simulink model "RMCHardwareInterfaceTUM_SiL"  (R2018b)
settings: configuration reference "Active" (kept outside this file)
undefined symbols (not defined in the file): PX2_Perception_IP_1, PX2_Perception_IP_2, PX2_Perception_IP_3, PX2_Perception_IP_4, PX2_Strategy_IP_1, PX2_Strategy_IP_2, PX2_Strategy_IP_3, PX2_Strategy_IP_4
libraries: dspnetwork x12
settings Model: DataDictionary=RMCHardwareInterfaceTUM_SiL.sldd  xpc_rtwmakecfg_data=_xpcetherlib__xpcether8255xlib__xpcetherGbElib__xpcnblib__xpciplib_  Creator=wischnewski  LastModifiedBy=ge34qer

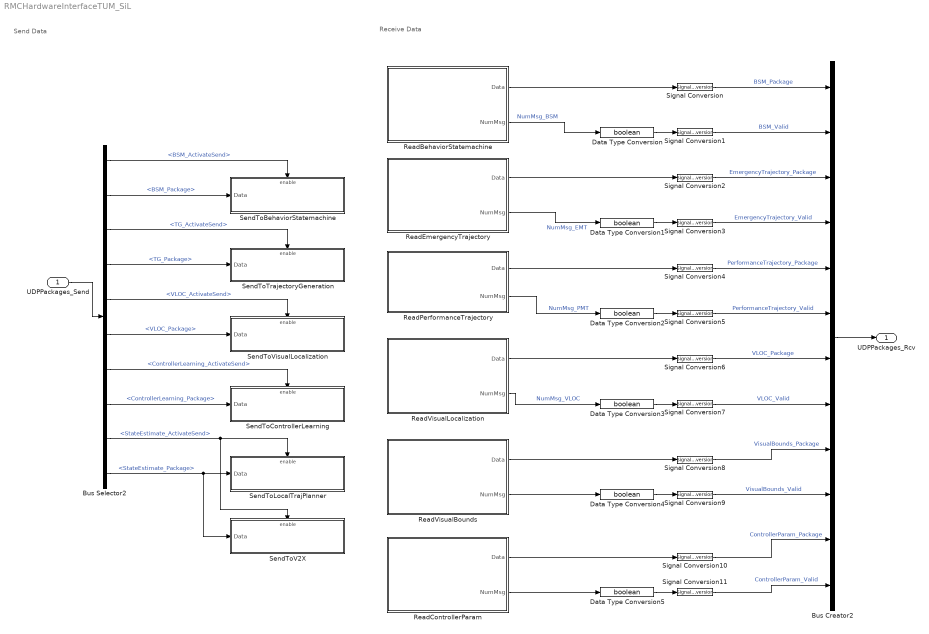
== system RMCHardwareInterfaceTUM_SiL ==
  note: Send Data
  note: Receive Data
  UDPPackages_Send : Inport  OutDataTypeStr=Bus: UDPPackages_Send
  Bus Creator2 : BusCreator  Inputs=12
  Bus Selector2 : BusSelector  OutputSignals=BSM_ActivateSend,BSM_Package,TG_ActivateSend,TG_Package,VLOC_ActivateSend,VLOC_Package,ControllerLearning_ActivateSend,ControllerLearning_Package,StateEstimate_ActivateSend,StateEstimate_Package
  Data Type Conversion{,1..5} (6 alike) : DataTypeConversion  OutDataTypeStr=boolean
  ReadBehaviorStatemachine : Subsystem  Priority=1000
  ReadControllerParam : Subsystem  Priority=1000
  ReadEmergencyTrajectory : Subsystem  Priority=1000
  ReadPerformanceTrajectory : Subsystem  Priority=1000
  ReadVisualBounds : Subsystem  Priority=1000
  ReadVisualLocalization : Subsystem  Priority=1000
  SendToBehaviorStatemachine : Subsystem
  SendToControllerLearning : Subsystem
  SendToLocalTrajPlanner : Subsystem
  SendToTrajectoryGeneration : Subsystem
  SendToV2X : Subsystem
  SendToVisualLocalization : Subsystem
  Signal Conversion{,1..11} (12 alike) : SignalConversion  OverrideOpt=off
  UDPPackages_Rcv : Outport  OutDataTypeStr=Bus: UDPPackages_Rcv
  wires:
  UDPPackages_Send/1 -> Bus Selector2/1
  Bus Selector2/2 -> SendToBehaviorStatemachine/1(Data)  "<BSM_Package>"
  Bus Selector2/1 -> SendToBehaviorStatemachine/Enable  "<BSM_ActivateSend>"
  Bus Selector2/4 -> SendToTrajectoryGeneration/1(Data)  "<TG_Package>"
  Bus Selector2/3 -> SendToTrajectoryGeneration/Enable  "<TG_ActivateSend>"
  Bus Selector2/6 -> SendToVisualLocalization/1(Data)  "<VLOC_Package>"
  Bus Selector2/5 -> SendToVisualLocalization/Enable  "<VLOC_ActivateSend>"
  Signal Conversion/1 -> Bus Creator2/1  "BSM_Package"
  Signal Conversion1/1 -> Bus Creator2/2  "BSM_Valid"
  Signal Conversion3/1 -> Bus Creator2/4  "EmergencyTrajectory_Valid"
  Signal Conversion2/1 -> Bus Creator2/3  "EmergencyTrajectory_Package"
  Signal Conversion4/1 -> Bus Creator2/5  "PerformanceTrajectory_Package"
  Signal Conversion5/1 -> Bus Creator2/6  "PerformanceTrajectory_Valid"
  Signal Conversion6/1 -> Bus Creator2/7  "VLOC_Package"
  Signal Conversion7/1 -> Bus Creator2/8  "VLOC_Valid"
  ReadVisualLocalization/1(Data) -> Signal Conversion6/1
  ReadBehaviorStatemachine/1(Data) -> Signal Conversion/1
  Data Type Conversion/1 -> Signal Conversion1/1
  ReadEmergencyTrajectory/1(Data) -> Signal Conversion2/1
  Data Type Conversion2/1 -> Signal Conversion5/1
  ReadPerformanceTrajectory/1(Data) -> Signal Conversion4/1
  Bus Creator2/1 -> UDPPackages_Rcv/1
  ReadBehaviorStatemachine/2(NumMsg) -> Data Type Conversion/1  "NumMsg_BSM"
  ReadEmergencyTrajectory/2(NumMsg) -> Data Type Conversion1/1  "NumMsg_EMT"
  ReadPerformanceTrajectory/2(NumMsg) -> Data Type Conversion2/1  "NumMsg_PMT"
  ReadVisualLocalization/2(NumMsg) -> Data Type Conversion3/1  "NumMsg_VLOC"
  Data Type Conversion1/1 -> Signal Conversion3/1
  Data Type Conversion3/1 -> Signal Conversion7/1
  ReadVisualBounds/1(Data) -> Signal Conversion8/1
  Data Type Conversion4/1 -> Signal Conversion9/1
  ReadVisualBounds/2(NumMsg) -> Data Type Conversion4/1
  Signal Conversion8/1 -> Bus Creator2/9  "VisualBounds_Package"
  Signal Conversion9/1 -> Bus Creator2/10  "VisualBounds_Valid"
  Data Type Conversion5/1 -> Signal Conversion11/1
  ReadControllerParam/1(Data) -> Signal Conversion10/1
  ReadControllerParam/2(NumMsg) -> Data Type Conversion5/1
  Signal Conversion10/1 -> Bus Creator2/11  "ControllerParam_Package"
  Signal Conversion11/1 -> Bus Creator2/12  "ControllerParam_Valid"
  Bus Selector2/7 -> SendToControllerLearning/Enable  "<ControllerLearning_ActivateSend>"
  Bus Selector2/8 -> SendToControllerLearning/1(Data)  "<ControllerLearning_Package>"
  Bus Selector2/10 -> SendToV2X/1(Data), SendToLocalTrajPlanner/1(Data)  "<StateEstimate_Package>"
  Bus Selector2/9 -> SendToV2X/Enable, SendToLocalTrajPlanner/Enable  "<StateEstimate_ActivateSend>"

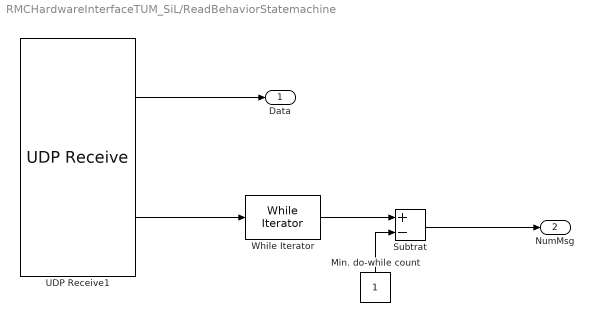
== system RMCHardwareInterfaceTUM_SiL/ReadBehaviorStatemachine ==
  Min. do-while count : Constant  OutDataTypeStr=int8
  Subtrat : Sum  Inputs=+-
  UDP Receive1 : dspnetwork/UDP Receive  localURL='0.0.0.0'  localPort=BehaviorStatemachineRcv_Port  remoteURL='0.0.0.0'  remotePort=-1  recvBufferSize=8192  dims=4  signalDatatype=uint8  isVarSize=off  showBlockingTime=on  blockingTime=0  sampletime=-1  blockPlatform=HOST
      settings: SourceProductName=DSP System Toolbox  SourceProductBaseCode=DS
  While Iterator : WhileIterator  MaxIters=-1  WhileBlockType=do-while  ShowIterationPort=on  OutputDataType=int16
  Data : Outport
  NumMsg : Outport  Port=2
  wires:
  While Iterator/1 -> Subtrat/1
  Min. do-while count/1 -> Subtrat/2
  Subtrat/1 -> NumMsg/1
  UDP Receive1/2 -> While Iterator/1
  UDP Receive1/1 -> Data/1

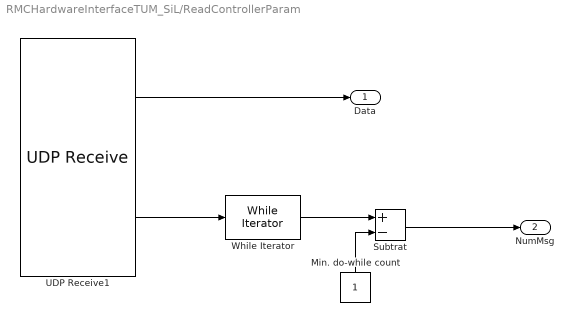
== system RMCHardwareInterfaceTUM_SiL/ReadControllerParam ==
  Min. do-while count : Constant  OutDataTypeStr=int8
  Subtrat : Sum  Inputs=+-
  UDP Receive1 : dspnetwork/UDP Receive  localURL='0.0.0.0'  localPort=ControllerParamRcv_Port  remoteURL='0.0.0.0'  remotePort=-1  recvBufferSize=8192  dims=1019  signalDatatype=uint8  isVarSize=off  showBlockingTime=on  blockingTime=0  sampletime=-1  blockPlatform=HOST
      settings: SourceProductName=DSP System Toolbox  SourceProductBaseCode=DS
  While Iterator : WhileIterator  MaxIters=-1  WhileBlockType=do-while  ShowIterationPort=on  OutputDataType=int16
  Data : Outport
  NumMsg : Outport  Port=2
  wires:
  UDP Receive1/2 -> While Iterator/1
  While Iterator/1 -> Subtrat/1
  Min. do-while count/1 -> Subtrat/2
  UDP Receive1/1 -> Data/1
  Subtrat/1 -> NumMsg/1

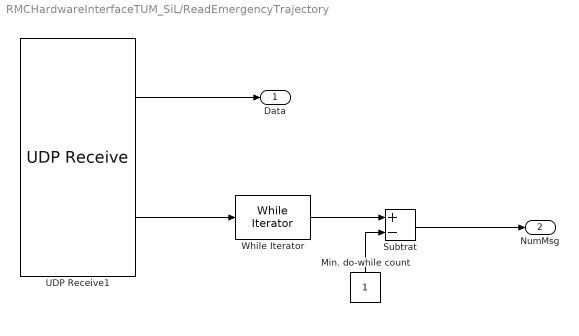
== system RMCHardwareInterfaceTUM_SiL/ReadEmergencyTrajectory ==
  Min. do-while count : Constant  OutDataTypeStr=int8
  Subtrat : Sum  Inputs=+-
  UDP Receive1 : dspnetwork/UDP Receive  localURL='0.0.0.0'  localPort=EmergencyPathRcv_Port  remoteURL='0.0.0.0'  remotePort=-1  recvBufferSize=8192  dims=1412  signalDatatype=uint8  isVarSize=off  showBlockingTime=on  blockingTime=0  sampletime=-1  blockPlatform=HOST
      settings: SourceProductName=DSP System Toolbox  SourceProductBaseCode=DS
  While Iterator : WhileIterator  MaxIters=-1  WhileBlockType=do-while  ShowIterationPort=on  OutputDataType=int16
  Data : Outport
  NumMsg : Outport  Port=2
  wires:
  While Iterator/1 -> Subtrat/1
  Min. do-while count/1 -> Subtrat/2
  UDP Receive1/2 -> While Iterator/1
  UDP Receive1/1 -> Data/1
  Subtrat/1 -> NumMsg/1

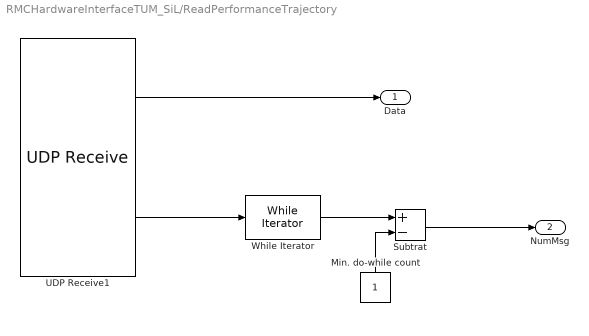
== system RMCHardwareInterfaceTUM_SiL/ReadPerformanceTrajectory ==
  Min. do-while count : Constant  OutDataTypeStr=int8
  Subtrat : Sum  Inputs=+-
  UDP Receive1 : dspnetwork/UDP Receive  localURL='0.0.0.0'  localPort=PerformanceTrajectoryRcv_Port  remoteURL='0.0.0.0'  remotePort=-1  recvBufferSize=8192  dims=1412  signalDatatype=uint8  isVarSize=off  showBlockingTime=on  blockingTime=0  sampletime=-1  blockPlatform=HOST
      settings: SourceProductName=DSP System Toolbox  SourceProductBaseCode=DS
  While Iterator : WhileIterator  MaxIters=-1  WhileBlockType=do-while  ShowIterationPort=on  OutputDataType=int16
  Data : Outport
  NumMsg : Outport  Port=2
  wires:
  UDP Receive1/2 -> While Iterator/1
  While Iterator/1 -> Subtrat/1
  Min. do-while count/1 -> Subtrat/2
  UDP Receive1/1 -> Data/1
  Subtrat/1 -> NumMsg/1

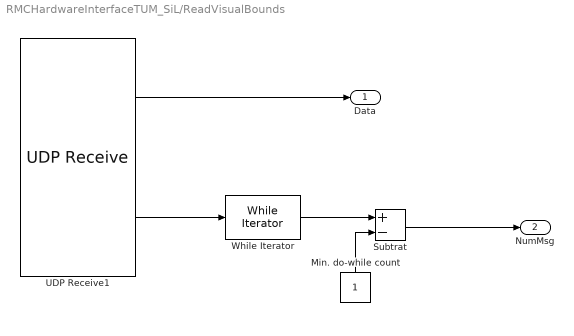
== system RMCHardwareInterfaceTUM_SiL/ReadVisualBounds ==
  Min. do-while count : Constant  OutDataTypeStr=int8
  Subtrat : Sum  Inputs=+-
  UDP Receive1 : dspnetwork/UDP Receive  localURL='0.0.0.0'  localPort=VisualBoundsRcv_Port  remoteURL='0.0.0.0'  remotePort=-1  recvBufferSize=8192  dims=24  signalDatatype=uint8  isVarSize=off  showBlockingTime=on  blockingTime=0  sampletime=-1  blockPlatform=HOST
      settings: SourceProductName=DSP System Toolbox  SourceProductBaseCode=DS
  While Iterator : WhileIterator  MaxIters=-1  WhileBlockType=do-while  ShowIterationPort=on  OutputDataType=int16
  Data : Outport
  NumMsg : Outport  Port=2
  wires:
  UDP Receive1/2 -> While Iterator/1
  While Iterator/1 -> Subtrat/1
  Min. do-while count/1 -> Subtrat/2
  UDP Receive1/1 -> Data/1
  Subtrat/1 -> NumMsg/1

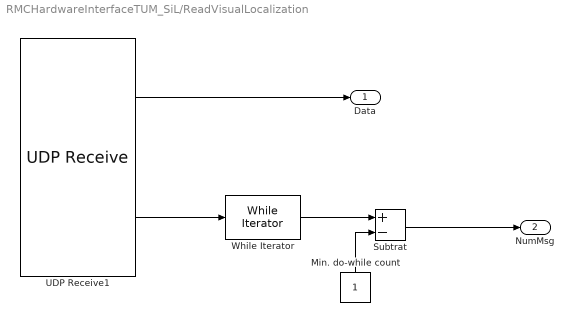
== system RMCHardwareInterfaceTUM_SiL/ReadVisualLocalization ==
  Min. do-while count : Constant  OutDataTypeStr=int8
  Subtrat : Sum  Inputs=+-
  UDP Receive1 : dspnetwork/UDP Receive  localURL='0.0.0.0'  localPort=VisualLocalizationRcv_Port  remoteURL='0.0.0.0'  remotePort=-1  recvBufferSize=8192  dims=48  signalDatatype=uint8  isVarSize=off  showBlockingTime=on  blockingTime=0  sampletime=-1  blockPlatform=HOST
      settings: SourceProductName=DSP System Toolbox  SourceProductBaseCode=DS
  While Iterator : WhileIterator  MaxIters=-1  WhileBlockType=do-while  ShowIterationPort=on  OutputDataType=int16
  Data : Outport
  NumMsg : Outport  Port=2
  wires:
  UDP Receive1/2 -> While Iterator/1
  While Iterator/1 -> Subtrat/1
  Min. do-while count/1 -> Subtrat/2
  UDP Receive1/1 -> Data/1
  Subtrat/1 -> NumMsg/1

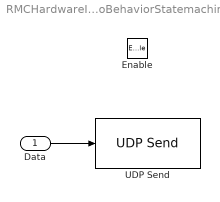
== system RMCHardwareInterfaceTUM_SiL/SendToBehaviorStatemachine ==
  Data : Inport
  Enable : EnablePort
  UDP Send : dspnetwork/UDP Send  remoteURL=[num2str(PX2_Strategy_IP_1) '.' num2str(PX2_Strategy_IP_2) '.' num2str(PX2_Strategy_IP_3) '.' num2str(PX2_Strategy_IP_4)]  remotePort=BehaviorStatemachineSend_Port  localURL='0.0.0.0'  localPortSource=Automatically determine  localPort=-1  sampletime=-1  blockPlatform=[]  separateLengthPort=0
      settings: SourceProductName=DSP System Toolbox  SourceProductBaseCode=DS
  wires:
  Data/1 -> UDP Send/1

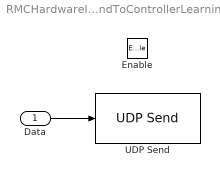
== system RMCHardwareInterfaceTUM_SiL/SendToControllerLearning ==
  Data : Inport
  Enable : EnablePort
  UDP Send : dspnetwork/UDP Send  remoteURL=[num2str(PX2_Strategy_IP_1) '.' num2str(PX2_Strategy_IP_2) '.' num2str(PX2_Strategy_IP_3) '.' num2str(PX2_Strategy_IP_4)]  remotePort=ControllerLearningSend_Port  localURL='0.0.0.0'  localPortSource=Automatically determine  localPort=-1  sampletime=-1  blockPlatform=[]  separateLengthPort=0
      settings: SourceProductName=DSP System Toolbox  SourceProductBaseCode=DS
  wires:
  Data/1 -> UDP Send/1

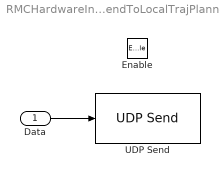
== system RMCHardwareInterfaceTUM_SiL/SendToLocalTrajPlanner ==
  Data : Inport
  Enable : EnablePort
  UDP Send : dspnetwork/UDP Send  remoteURL=[num2str(PX2_Strategy_IP_1) '.' num2str(PX2_Strategy_IP_2) '.' num2str(PX2_Strategy_IP_3) '.' num2str(PX2_Strategy_IP_4)]  remotePort=LocalTrajPlannerSend_Port  localURL='0.0.0.0'  localPortSource=Automatically determine  localPort=-1  sampletime=-1  blockPlatform=[]  separateLengthPort=0
      settings: SourceProductName=DSP System Toolbox  SourceProductBaseCode=DS
  wires:
  Data/1 -> UDP Send/1

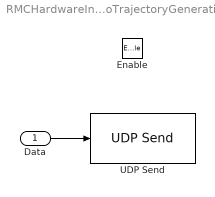
== system RMCHardwareInterfaceTUM_SiL/SendToTrajectoryGeneration ==
  Data : Inport
  Enable : EnablePort
  UDP Send : dspnetwork/UDP Send  remoteURL=[num2str(PX2_Strategy_IP_1) '.' num2str(PX2_Strategy_IP_2) '.' num2str(PX2_Strategy_IP_3) '.' num2str(PX2_Strategy_IP_4)]  remotePort=TrajectoryGenerationSend_Port  localURL='0.0.0.0'  localPortSource=Automatically determine  localPort=-1  sampletime=-1  blockPlatform=[]  separateLengthPort=0
      settings: SourceProductName=DSP System Toolbox  SourceProductBaseCode=DS
  wires:
  Data/1 -> UDP Send/1

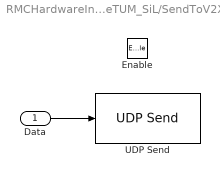
== system RMCHardwareInterfaceTUM_SiL/SendToV2X ==
  Data : Inport
  Enable : EnablePort
  UDP Send : dspnetwork/UDP Send  remoteURL=[num2str(PX2_Perception_IP_1) '.' num2str(PX2_Perception_IP_2) '.' num2str(PX2_Perception_IP_3) '.' num2str(PX2_Perception_IP_4)]  remotePort=V2XSend_Port  localURL='0.0.0.0'  localPortSource=Automatically determine  localPort=-1  sampletime=-1  blockPlatform=[]  separateLengthPort=0
      settings: SourceProductName=DSP System Toolbox  SourceProductBaseCode=DS
  wires:
  Data/1 -> UDP Send/1

== system RMCHardwareInterfaceTUM_SiL/SendToVisualLocalization ==
  Data : Inport
  Enable : EnablePort
  UDP Send : dspnetwork/UDP Send  remoteURL=[num2str(PX2_Perception_IP_1) '.' num2str(PX2_Perception_IP_2) '.' num2str(PX2_Perception_IP_3) '.' num2str(PX2_Perception_IP_4)]  remotePort=VisualLocalizationSend_Port  localURL='0.0.0.0'  localPortSource=Automatically determine  localPort=-1  sampletime=-1  blockPlatform=[]  separateLengthPort=0
      settings: SourceProductName=DSP System Toolbox  SourceProductBaseCode=DS
  wires:
  Data/1 -> UDP Send/1
